simulink model "model"  (R2021b)
settings: Solver=VariableStepAuto  StartTime=0.0  StopTime=1175  RelTol=1e-3
values from neighbouring files (symbols this model uses):
  capacity_batt = 8    [init.m]    (also in workspace.mat = 10.5)
  Cr = 0.013    [datavehicule.m]    (also in workspace.mat)
  Cx = 0.25    [datavehicule.m]    (also in workspace.mat)
  epsilon = 10^-6    (= 1e-06)    [init.m]
  final_drive = 4.125    [init.m]
  g = 9.81    [datavehicule.m]    (also in init.m; workspace.mat)
  Gear_ratio = 0.89    [init.m]    (also in workspace.mat = 0.111111111111)
  gr = 17/64    (= 0.265625)    [datavehicule.m]    (also in workspace.mat)
  M = 1400    [datavehicule.m]    (also in workspace.mat)
  p = 0    [datavehicule.m]    (also in workspace.mat)
  power_FC_max = 45    [workspace.mat]
  ro = 1.23    [datavehicule.m]    (also in workspace.mat)
  V = [t, velocity]    [init.m]
  wheel_radius = 0.29    [workspace.mat]
undefined symbols (not defined in the file or in its folder): DiscIntNeverNeededParam, Ion, Lithium, Ts
libraries: sdl_lib x8, spsCurrentMeasurementLib x6, fl_lib x6, nesl_utility x6, spsSeriesRLCBranchLib x4, AC6DriveInternalModels x3, simulink x2, spsBatteryLib x1, simulink_extras x1, DC6DriveInternalModels x1, spsDiodeLib x1, spsFuelCellStackLib x1
(part 2 of 2)

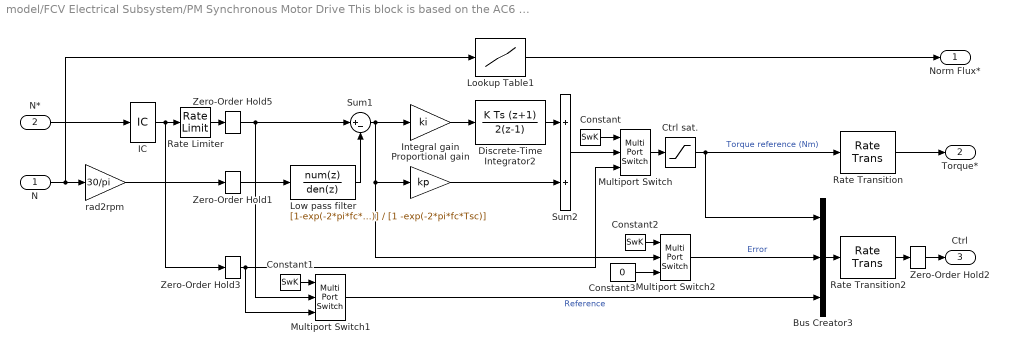
== system model/FCV Electrical Subsystem/PM Synchronous Motor Drive This block is based on the AC6 drive block/Speed Controller ==
  N : Inport
  N* : Inport  Port=2
  Bus Creator3 : BusCreator  Inputs=3
  Constant : Constant  Value=SwK
  Constant1 : Constant  Value=SwK
  Constant2 : Constant  Value=SwK
  Constant3 : Constant  Value=0
  Ctrl sat. : Saturate  UpperLimit=ctrl_sat(2)  LowerLimit=ctrl_sat(1)
  Discrete-Time Integrator2 : DiscreteIntegrator  IntegratorMethod=Integration: Trapezoidal  SampleTime=Tsc  LimitOutput=on  UpperSaturationLimit=ctrl_sat(2)  LowerSaturationLimit=ctrl_sat(1)  ICPrevOutput=DiscIntNeverNeededParam  ICPrevScaledInput=DiscIntNeverNeededParam
  IC : InitialCondition  Value=0
  Integral gain : Gain  Gain=ki  SaturateOnIntegerOverflow=on  OutDataTypeStr=Inherit: Same as input  ParamDataTypeStr=Inherit: Same as input
  Lookup Table1 : Lookup  InputValues=[0 38 40 45 50 60 80 100 120 140 160]*(12500/160/30*pi)  Table="[1 1 0.92 0.86 .83  0.78 0.71 0.675 0.652 0.637 0.612]"
  Low pass filter : DiscreteTransferFcn  Numerator=[1-exp(-2*pi*fc*Tsc)]  Denominator=[1 -exp(-2*pi*fc*Tsc)]  SampleTime=Tsc
  Multiport Switch : MultiPortSwitch  Inputs=2  SaturateOnIntegerOverflow=on
  Multiport Switch1 : MultiPortSwitch  Inputs=2  SaturateOnIntegerOverflow=on
  Multiport Switch2 : MultiPortSwitch  Inputs=2  SaturateOnIntegerOverflow=on
  Proportional gain : Gain  Gain=kp  SaturateOnIntegerOverflow=on  OutDataTypeStr=Inherit: Same as input  ParamDataTypeStr=Inherit: Same as input
  Rate Limiter : RateLimiter  RisingSlewLimit=ramp(2)  FallingSlewLimit=ramp(1)  LinearizeAsGain=off
  Rate Transition : RateTransition
  Rate Transition2 : RateTransition
  Sum1 : Sum  Inputs=|+-  InputSameDT=on  SaturateOnIntegerOverflow=on  OutDataTypeStr=Inherit: Same as first input
  Sum2 : Sum  InputSameDT=on  SaturateOnIntegerOverflow=on  OutDataTypeStr=Inherit: Same as first input
  Zero-Order Hold1 : ZeroOrderHold  SampleTime=Tsc
  Zero-Order Hold2 : ZeroOrderHold  SampleTime=Ts
  Zero-Order Hold3 : ZeroOrderHold  SampleTime=Tsc
  Zero-Order Hold5 : ZeroOrderHold  SampleTime=Tsc
  rad2rpm : Gain  Gain=30/pi  SaturateOnIntegerOverflow=on  OutDataTypeStr=Inherit: Same as input  ParamDataTypeStr=Inherit: Same as input
  Norm Flux* : Outport
  Torque* : Outport  Port=2
  Ctrl : Outport  Port=3
  wires:
  Lookup Table1/1 -> Norm Flux*/1
  rad2rpm/1 -> Zero-Order Hold1/1
  N*/1 -> IC/1
  Ctrl sat./1 -> Rate Transition/1, Bus Creator3/1  "Torque reference (Nm)"
  Integral gain/1 -> Discrete-Time Integrator2/1
  Sum1/1 -> Integral gain/1, Proportional gain/1, Multiport Switch2/2
  N/1 -> Lookup Table1/1, rad2rpm/1
  Discrete-Time Integrator2/1 -> Sum2/1
  Proportional gain/1 -> Sum2/2
  Rate Transition/1 -> Torque*/1
  IC/1 -> Rate Limiter/1, Zero-Order Hold3/1
  Zero-Order Hold1/1 -> Low pass filter/1
  Rate Transition2/1 -> Zero-Order Hold2/1
  Bus Creator3/1 -> Rate Transition2/1
  Zero-Order Hold2/1 -> Ctrl/1
  Low pass filter/1 -> Sum1/2
  Rate Limiter/1 -> Zero-Order Hold5/1
  Zero-Order Hold5/1 -> Sum1/1, Multiport Switch1/2
  Multiport Switch/1 -> Ctrl sat./1
  Constant/1 -> Multiport Switch/1
  Sum2/1 -> Multiport Switch/2
  Constant1/1 -> Multiport Switch1/1
  Zero-Order Hold3/1 -> Multiport Switch/3, Multiport Switch1/3
  Multiport Switch1/1 -> Bus Creator3/3  "Reference"
  Multiport Switch2/1 -> Bus Creator3/2  "Error"
  Constant2/1 -> Multiport Switch2/1
  Constant3/1 -> Multiport Switch2/3

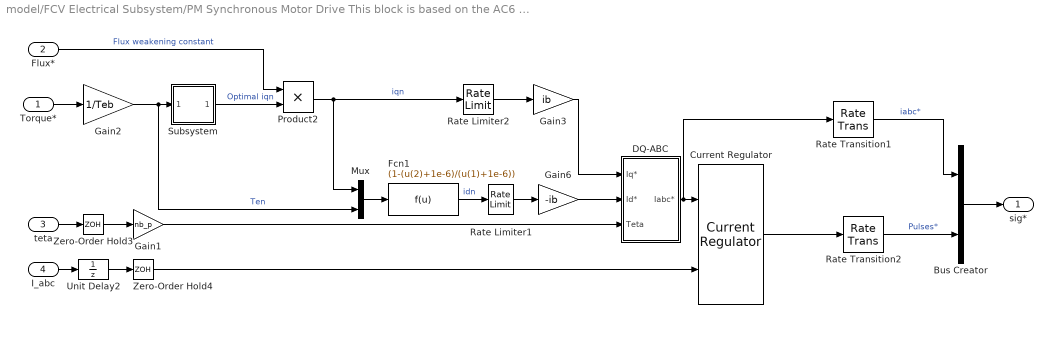
== system model/FCV Electrical Subsystem/PM Synchronous Motor Drive This block is based on the AC6 drive block/VECT ==
  Torque* : Inport
  Flux* : Inport  Port=2
  teta : Inport  Port=3
  I_abc : Inport  Port=4
  Bus Creator : BusCreator  Inputs=2
  Current Regulator : AC6DriveInternalModels/VECT (average model)/Current Regulator  SystemSampleTime=-1  VariantActivationTime=update diagram  Latency=0  AutoFrameSizeCalculation=off
      settings: SourceProductBaseCode=PS
  DQ-ABC : Subsystem
  Fcn1 : Fcn  Expr=(1-(u(2)+1e-6)/(u(1)+1e-6))
  Gain1 : Gain  Gain=nb_p  SaturateOnIntegerOverflow=on  OutDataTypeStr=Inherit: Same as input  ParamDataTypeStr=Inherit: Same as input
  Gain2 : Gain  Gain=1/Teb  SaturateOnIntegerOverflow=on  OutDataTypeStr=Inherit: Same as input  ParamDataTypeStr=Inherit: Same as input
  Gain3 : Gain  Gain=ib  SaturateOnIntegerOverflow=on  OutDataTypeStr=Inherit: Same as input  ParamDataTypeStr=Inherit: Same as input
  Gain6 : Gain  Gain=-ib  SaturateOnIntegerOverflow=on  OutDataTypeStr=Inherit: Same as input  ParamDataTypeStr=Inherit: Same as input
  Mux : Mux  Inputs=2
  Product2 : Product  RndMeth=Zero
  Rate Limiter1 : RateLimiter  RisingSlewLimit=500  FallingSlewLimit=-500  SampleTimeMode=inherited
  Rate Limiter2 : RateLimiter  RisingSlewLimit=500  FallingSlewLimit=-500  SampleTimeMode=inherited
  Rate Transition1 : RateTransition
  Rate Transition2 : RateTransition
  Subsystem : Subsystem
  Unit Delay2 : UnitDelay  SampleTime=-1  HasFrameUpgradeWarning=on
  Zero-Order Hold3 : ZeroOrderHold  SampleTime=Ts_vect
  Zero-Order Hold4 : ZeroOrderHold  SampleTime=Ts_vect
  sig* : Outport
  wires:
  Rate Limiter1/1 -> Gain6/1
  Rate Limiter2/1 -> Gain3/1
  Gain3/1 -> DQ-ABC/1("Iq* ")
  Rate Transition1/1 -> Bus Creator/1  "iabc*"
  Rate Transition2/1 -> Bus Creator/2  "Pulses*"
  Bus Creator/1 -> sig*/1
  Subsystem/1(iqn) -> Product2/2  "Optimal iqn"
  Product2/1 -> Rate Limiter2/1, Mux/1  "iqn"
  Fcn1/1 -> Rate Limiter1/1  "idn"
  Gain6/1 -> DQ-ABC/2("Id* ")
  Flux*/1 -> Product2/1  "Flux weakening constant"
  Mux/1 -> Fcn1/1
  Gain2/1 -> Mux/2, Subsystem/1(Ten)  "Ten"
  Torque*/1 -> Gain2/1
  I_abc/1 -> Unit Delay2/1
  DQ-ABC/1(Iabc*) -> Current Regulator/1, Rate Transition1/1
  Gain1/1 -> DQ-ABC/3(Teta)
  Zero-Order Hold3/1 -> Gain1/1
  teta/1 -> Zero-Order Hold3/1
  Current Regulator/1 -> Rate Transition2/1
  Zero-Order Hold4/1 -> Current Regulator/2
  Unit Delay2/1 -> Zero-Order Hold4/1

== system model/FCV Electrical Subsystem/DC-DC converter/Bus DC controller/Current controller DISCRETE1 ==
  ifc : Inport
  iref : Inport  Port=2
  Ctrl sat. : Saturate  UpperLimit=0.95  LowerLimit=-0.95
  Discrete-Time Integrator : DiscreteIntegrator  IntegratorMethod=Integration: Trapezoidal  SampleTime=Ts  LimitOutput=on  UpperSaturationLimit=1  LowerSaturationLimit=-1  ICPrevOutput=DiscIntNeverNeededParam  ICPrevScaledInput=DiscIntNeverNeededParam
  Integral gain : Gain  Gain=Ki  SaturateOnIntegerOverflow=on  OutDataTypeStr=Inherit: Same as input  ParamDataTypeStr=Inherit: Same as input
  Proportional gain : Gain  Gain=Kp  SaturateOnIntegerOverflow=on  OutDataTypeStr=Inherit: Same as input  ParamDataTypeStr=Inherit: Same as input
  Sum1 : Sum  Inputs=+-  InputSameDT=on  SaturateOnIntegerOverflow=on  OutDataTypeStr=Inherit: Same as first input
  Sum2 : Sum  InputSameDT=on  SaturateOnIntegerOverflow=on  OutDataTypeStr=Inherit: Same as first input
  Ec : Outport  InitialOutput=0
  wires:
  Proportional gain/1 -> Sum2/1
  Integral gain/1 -> Discrete-Time Integrator/1
  Sum1/1 -> Integral gain/1, Proportional gain/1
  ifc/1 -> Sum1/1
  iref/1 -> Sum1/2
  Discrete-Time Integrator/1 -> Sum2/2
  Sum2/1 -> Ctrl sat./1
  Ctrl sat./1 -> Ec/1

== system model/FCV Electrical Subsystem/DC-DC converter/Bus DC controller/Duty Cycles ==
  Ec : Inport
  Add : Sum  Inputs=+-
  Bus Creator2 : BusCreator  Inputs=2
  Constant : Constant
  Duty Cycle : Fcn  Expr=0.5*(u[1]+1)
  dc : Outport
  wires:
  Add/1 -> Bus Creator2/1  "IGBT 2"
  Duty Cycle/1 -> Bus Creator2/2, Add/2  "IGBT I"
  Constant/1 -> Add/1
  Ec/1 -> Duty Cycle/1
  Bus Creator2/1 -> dc/1

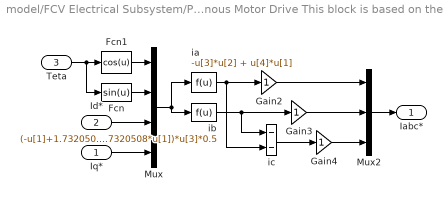
== system model/FCV Electrical Subsystem/PM Synchronous Motor Drive This block is based on the AC6 drive block/VECT/DQ-ABC ==
  "Iq* " : Inport
  "Id* " : Inport  Port=2
  Teta : Inport  Port=3
  Fcn : Fcn  Expr=sin(u)
  Fcn1 : Fcn  Expr=cos(u)
  Gain2 : Gain  SaturateOnIntegerOverflow=on  OutDataTypeStr=Inherit: Same as input  ParamDataTypeStr=Inherit: Same as input
  Gain3 : Gain  SaturateOnIntegerOverflow=on  OutDataTypeStr=Inherit: Same as input  ParamDataTypeStr=Inherit: Same as input
  Gain4 : Gain  SaturateOnIntegerOverflow=on  OutDataTypeStr=Inherit: Same as input  ParamDataTypeStr=Inherit: Same as input
  Mux : Mux
  Mux2 : Mux  Inputs=3
  ia : Fcn  Expr=-u[3]*u[2] + u[4]*u[1]
  ib : Fcn  Expr=(-u[1]+1.7320508*u[2])*u[4]*0.5+(u[2]+1.7320508*u[1])*u[3]*0.5
  ic : Sum  Inputs=--  InputSameDT=on  SaturateOnIntegerOverflow=on  OutDataTypeStr=Inherit: Same as first input
  Iabc* : Outport  InitialOutput=0
  wires:
  ib/1 -> ic/1, Gain3/1
  ia/1 -> ic/2, Gain2/1
  Gain2/1 -> Mux2/1
  Gain4/1 -> Mux2/3
  ic/1 -> Gain4/1
  Gain3/1 -> Mux2/2
  "Iq* "/1 -> Mux/4
  "Id* "/1 -> Mux/3
  Teta/1 -> Fcn/1, Fcn1/1
  Mux/1 -> ia/1, ib/1
  Mux2/1 -> Iabc*/1
  Fcn1/1 -> Mux/1
  Fcn/1 -> Mux/2

== system model/FCV Electrical Subsystem/PM Synchronous Motor Drive This block is based on the AC6 drive block/VECT/Subsystem ==
  Ten : Inport
  Abs : Abs
  Fcn2 : Fcn  Expr=(sqrt(4*0.5*u(1)+1)-1)/(2*0.5)
  Product1 : Product  RndMeth=Zero
  Sign : Signum
  iqn : Outport
  wires:
  Product1/1 -> iqn/1
  Ten/1 -> Sign/1, Abs/1
  Sign/1 -> Product1/2
  Fcn2/1 -> Product1/1
  Abs/1 -> Fcn2/1

== matlab function model/Rendement/MATLAB Function ==
  data: power input; power_transmission output
function power_transmission = transmission_eff(power)

    power_transmission = power*(1/0.98);
end

== matlab function model/MATLAB Function ==
  data: time input; Ft output; velocity input; acceleration input; Facc output; Froul output; Fprof output; Faero output; Force_parameters input
function [ Ft, Facc, Froul , Fprof, Faero ] = ForceTrac( time, velocity,acceleration,Force_parameters  )
% Calcule les forces necessaires au déplacement d'un vehicule
% time est en sec
% velocity est en m/s
% le vecteur time et velocity ont la même taille et doivent avoir au
% minimum 2 colonnes
Cr,Cx,g,gr,M,p,ro = Force_parameters.Cr,Force_parameters.Cx,Force_parameters.g,Force_parameters.gr,Force_parameters.M,Force_parameters.p,Force_parameters.ro
[l c]=size(time);
if l>c              % inversion des lignes et des colonnes 
   time=time';
   velocity=velocity'
end
[l c]=size(time);


% Equations mecanique
delta=1.04+0.0025*gr^2;
Facc=delta.*M.*acceleration; % .* multiplication terme à terme
Froul=(M.*g.*Cr).*ones(1,c);
Fprof=M.*g.*sin(atan(p)).*ones(1,c);
  Sf=1.6+0.00056*(M-765);
Faero=0.5*ro*Cx*Sf.*velocity.^2;

Ft=Facc+Froul+Fprof+Faero;

% % test
% % 50km/h = 50*1000/3600m/s
% [ Ft Facc Froul Fprof Faero ] = ForceTrac( [0, 10], [50*1000/3600, 50*1000/3600] )
% [ Ft Facc Froul Fprof Faero ] = ForceTrac( [0, 10], [0*1000/3600, 100*1000/3600] )
% [ Ft Facc Froul Fprof Faero ] = ForceTrac( cycle.Time, cycle.Speed.*1000/3600 )

end

== matlab function model/Rendement/MATLAB Function1 ==
  data: power input; power_motor output
function power_motor = motor_eff(power)

    power_motor = power*(1/0.89);
end

== matlab function model/Rendement/MATLAB Function2 ==
  data: power input; power_battery output
function power_battery = battery_eff(power)

    power_battery = power*(1/0.95);
end

== matlab function model/Rendement/MATLAB Function3 ==
  data: power input; power_fuel_cell output
function power_fuel_cell = fuel_cell_eff(power)

    power_fuel_cell = power*(1/0.53);
end

== matlab function model/H2 comsuption ==
  data: energy_FC input; H2_consuption output
function H2_consuption = fcn(energy_FC)
%calculate the hydrogen consumption in grams, knowing that that the energy density of
%hydrogen is 142MJ/kg which is equal to 142,000J/g
%a reverifier

 H2_consuption= energy_FC./142000;

end

== matlab function model/Rendement/MATLAB Function4 ==
  data: power_motor input; power_battery output; power_FC_max input; need_battery input; power_FC output
function [power_battery,power_FC]= trans_eff(power_motor,power_FC_max,need_battery)

    if need_battery == true
            power_battery =  (power_motor - power_FC_max)*(1/0.90);

            power_FC = power_FC_max;

        
    else
            power_FC = power_motor;
            power_battery = 0;

        
  
end

== matlab function model/motor speed calculation/MATLAB Function ==
  data: motor_speed input; motor_speed_rpm output
function motor_speed_rpm = fcn(motor_speed)

motor_speed_rpm = motor_speed*60/(2*pi);
